simulink model "slexRegressionGPPredictExample"  (R2023a)
settings: Solver=FixedStepDiscrete  StartTime=0.0  StopTime=modelInput.time(end)  RelTol=1e-3
PreLoadFcn:
  | if ~exist("gpMdl","var")
  | 
  | load gprdata
  | gpMdl = fitrgp(Xtrain,ytrain,Standardize=1);
  | modelInput.time = (0:length(ytest)-1)';
  | modelInput.signals(1).values = Xtest;
  | modelInput.signals(1).dimensions = size(Xtest,2);
  | 
  | end
values from neighbouring files (symbols this model uses):
  ytest = [283.168893324 278.954933977 277.364283814 279.890559023 279.903214995 278.639437691 290.001035622 285.377237967 280.214912093 289.869498081 283.444297371 282.718089302 ... (100 elements, 100x1)]    [gprdata.mat]
libraries: statsLibrary x1
settings Model: Creator=The MathWorks, Inc.  LastModifiedBy=The MathWorks, Inc.
settings SolverCC: MaxZcPerStep=1
settings DataIOCC: ExternalInput=modelInput  LoadExternalInput=on
settings ModelReferenceCC: EnableRefExpFcnMdlSchedulingChecks=on
settings RTWCC: DLArmComputeVersion=19.05

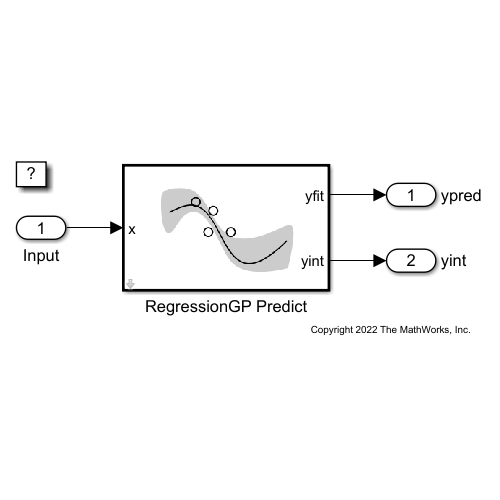
[thumbnail: Simulink's stored preview of the top-level diagram]
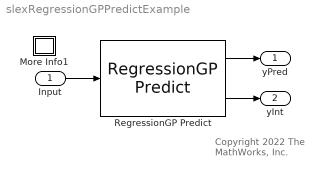
== system slexRegressionGPPredictExample ==
  note: Copyright 2022 The MathWorks, Inc.
  Input : Inport  PortDimensions=6  SampleTime=1
  More Info1 : Subsystem
      settings: OpenFcn=showExample('stats/PredictResponsesUsingRegressionGPPredictBlockExample')
      mask Display: disp('?')
  RegressionGP Predict : statsLibrary/Regression/RegressionGP Predict  TrainedLearner=gpMdl  ShowOutputSD=off  ShowOutputIntervals=on  Alpha=0.05  OutMin=[]  OutMax=[]  SDOutMin=[]  SDOutMax=[]  IntervalsOutMin=[]  IntervalsOutMax=[]  KernelMin=[]  KernelMax=[]  DistanceOutMin=[]  DistanceOutMax=[]  BasisOutMin=[]  BasisOutMax=[]  StandardizedInputOutMin=[]  StandardizedInputOutMax=[]  KernelParam1Min=[]  KernelParam1Max=[]  KernelParam2Min=[]  KernelParam2Max=[]  KernelParam3Min=[]  KernelParam3Max=[]  KernelParam4Min=[]  KernelParam4Max=[]  BasisParam1Min=[]  BasisParam1Max=[]  BasisParam2Min=[]  BasisParam2Max=[]  SDParam1Min=[]  SDParam1Max=[]  KernelParam5Min=[]  KernelParam5Max=[]
  yPred : Outport  SignalName=ypred
  yInt : Outport  Port=2  SignalName=yint
  wires:
  Input/1 -> RegressionGP Predict/1
  RegressionGP Predict/1 -> yPred/1
  RegressionGP Predict/2 -> yInt/1

== system slexRegressionGPPredictExample/More Info1 ==
